simulink model "RecurDyn_Client_Block_9_1"  (R2018b)
settings: Solver=ode45  StartTime=0.0  StopTime=1.0  FixedStep=Control_timestep  RelTol=1e-3  AbsTol=1e-6
values from neighbouring files (symbols this model uses):
  Matlab_version = str2double(r_temp___(1))    [quadruped.m]
  Output_File = 'quadruped_demo1'    [quadruped.m]
  Output_file_n = r_temp___(2)    [quadruped.m]
  Plant_inputs_num = r_temp___(1)    [quadruped.m]
  Plant_outputs_num = r_temp___(1)    [quadruped.m]
  RecurDyn = 'C:\Program Files\FunctionBay, Inc\RecurDyn V9R1\Bin\'    [quadruped.m]
  RecurDyn_controltimestep = 1.e-003    (= 0.001)    [quadruped.m]
  RecurDyn_model = 'quadruped_demo1'    [quadruped.m]
  RecurDyn_model_n = r_temp___(2)    [quadruped.m]
settings Model: ExtModeTrigMode=oneshot  ExtModeArmWhenConnect=off  Creator=hgildong  LastModifiedBy=ahl19
settings SolverCC: AutoScaleAbsTol=off
settings DataIOCC: SaveFormat=Array  SignalLoggingSaveFormat=ModelDataLogs
settings OptimizationCC: BooleanDataType=off  ExpressionDepthLimit=2147483647  InitFltsAndDblsToZero=on  LifeSpan=inf
settings DebuggingCC: SaveWithParameterizedLinksMsg=none  UnderspecifiedInitializationDetection=Classic  MergeDetectMultiDrivingBlocksExec=none  SignalResolutionControl=TryResolveAllWithWarning  MultiTaskDSMMsg=warning  MultiTaskCondExecSysMsg=none  FcnCallInpInsideContextMsg=warning  StateNameClashWarn=warning  SFUnexpectedBacktrackingDiag=warning  SFNoUnconditionalDefaultTransitionDiag=warning  SFExecutionAtInitializationDiag=none
settings HardwareCC: ProdBitPerPointer=32  ProdBitPerSizeT=32  ProdBitPerPtrDiffT=32  ProdLargestAtomicFloat=None  ProdIntDivRoundTo=Undefined  ProdEndianess=Unspecified  ProdWordSize=32  ProdHWDeviceType=32-bit Generic  TargetUnknown=on
settings ModelReferenceCC: PropagateSignalLabelsOutOfModel=off
settings SFSimCC: SimUseLocalCustomCode=off
settings RTWCC: TemplateMakefile=grt_unix.tmf  RTWUseLocalCustomCode=off
settings CodeAppCC: StateflowObjectComments=on
settings GRTTargetCC: TargetFcnLib=ansi_tfl_tmw.mat  TargetLangStandard=C89/C90 (ANSI)  ModelReferenceCompliant=off  GeneratePreprocessorConditionals=Disable all  CombineOutputUpdateFcns=off  MatFileLogging=off  GRTInterface=on
settings ConfigComp: CovMetricSettings=dw  CovHtmlReporting=on  CovSaveCumulativeToWorkspaceVar=on  CovSaveSingleToWorkspaceVar=on  CovExternalEMLEnable=off

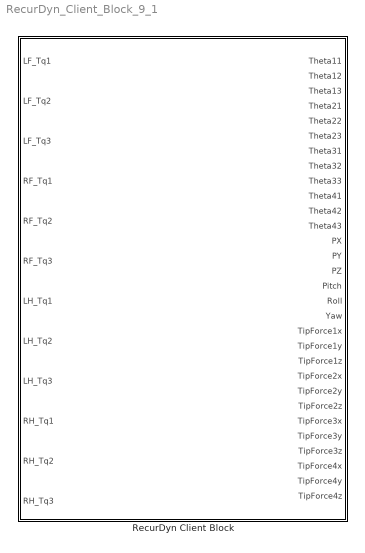
== system RecurDyn_Client_Block_9_1 ==
  RecurDyn Client Block : Subsystem
      mask Display: image(imread('RecurDyn_IF3x_Client.jpg'))

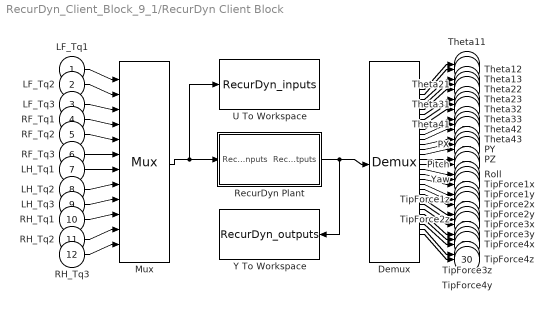
== system RecurDyn_Client_Block_9_1/RecurDyn Client Block ==
  LF_Tq1 : Inport
  LF_Tq2 : Inport  Port=2
  LF_Tq3 : Inport  Port=3
  RF_Tq1 : Inport  Port=4
  RF_Tq2 : Inport  Port=5
  RF_Tq3 : Inport  Port=6
  LH_Tq1 : Inport  Port=7
  LH_Tq2 : Inport  Port=8
  LH_Tq3 : Inport  Port=9
  RH_Tq1 : Inport  Port=10
  RH_Tq2 : Inport  Port=11
  RH_Tq3 : Inport  Port=12
  Demux : Demux  Outputs=30
  Mux : Mux  Inputs=12
  RecurDyn Plant : Subsystem  mask(Recurdyn/Plant){RecurDyn_model_name=RecurDyn_model, Output_File_Name_=Output_File, RecurDyn_=RecurDyn, Matlab_version_=Matlab_version, RecurDyn_controltimestep_=RecurDyn_controltimestep, RecurDyn_step_=100, Waitingtime=1000, RecurDyn_static_=off, RecurDyn_show_=on, RecurDyn_ani_=on, Create_Output_Folder_=off}
      mask prompts: Output_File_Name_ "Output File Name"; RecurDyn_ "RecurDyn_install_directory"; Matlab_version_ "Matlab version"; RecurDyn_controltimestep_ "Sampling period"; RecurDyn_step_ "RecurDyn_step"; Waitingtime "Waiting time"; RecurDyn_static_ "Static analysis"; RecurDyn_show_ "RecurDyn_show"; RecurDyn_ani_ "RecurDyn_animation"; Create_Output_Folder_ "Create Output Folder"
      mask help:
      | Simulate any Recurdyn Dynamics Model in Recurdyn/Solver
      | Plant inputs and Plant outputs are transfered every sampling time
      | Here, sampling time is determined by sampling period (Control time step)
      mask Display: disp( 'Dynamic Model' )
  U To Workspace : ToWorkspace  VariableName=RecurDyn_inputs
  Y To Workspace : ToWorkspace  VariableName=RecurDyn_outputs
  "Theta11   " : Outport
  "Theta12   " : Outport  Port=2
  "Theta13   " : Outport  Port=3
  "Theta21   " : Outport  Port=4
  "Theta22   " : Outport  Port=5
  "Theta23   " : Outport  Port=6
  "Theta31   " : Outport  Port=7
  "Theta32   " : Outport  Port=8
  "Theta33   " : Outport  Port=9
  "Theta41   " : Outport  Port=10
  "Theta42   " : Outport  Port=11
  "Theta43   " : Outport  Port=12
  "PX        " : Outport  Port=13
  "PY        " : Outport  Port=14
  "PZ        " : Outport  Port=15
  "Pitch     " : Outport  Port=16
  "Roll      " : Outport  Port=17
  "Yaw       " : Outport  Port=18
  TipForce1x : Outport  Port=19
  TipForce1y : Outport  Port=20
  TipForce1z : Outport  Port=21
  TipForce2x : Outport  Port=22
  TipForce2y : Outport  Port=23
  TipForce2z : Outport  Port=24
  TipForce3x : Outport  Port=25
  TipForce3y : Outport  Port=26
  TipForce3z : Outport  Port=27
  TipForce4x : Outport  Port=28
  TipForce4y : Outport  Port=29
  TipForce4z : Outport  Port=30
  wires:
  RecurDyn Plant/1(RecurDyn_outputs) -> Demux/1, Y To Workspace/1
  Mux/1 -> RecurDyn Plant/1(" RecurDyn_inputs"), U To Workspace/1
  Demux/1 -> "Theta11   "/1
  Demux/2 -> "Theta12   "/1
  Demux/3 -> "Theta13   "/1
  Demux/4 -> "Theta21   "/1
  Demux/5 -> "Theta22   "/1
  Demux/6 -> "Theta23   "/1
  Demux/7 -> "Theta31   "/1
  Demux/8 -> "Theta32   "/1
  Demux/9 -> "Theta33   "/1
  Demux/10 -> "Theta41   "/1
  Demux/11 -> "Theta42   "/1
  Demux/12 -> "Theta43   "/1
  Demux/13 -> "PX        "/1
  Demux/14 -> "PY        "/1
  Demux/15 -> "PZ        "/1
  Demux/16 -> "Pitch     "/1
  Demux/17 -> "Roll      "/1
  Demux/18 -> "Yaw       "/1
  Demux/19 -> TipForce1x/1
  Demux/20 -> TipForce1y/1
  Demux/21 -> TipForce1z/1
  Demux/22 -> TipForce2x/1
  Demux/23 -> TipForce2y/1
  Demux/24 -> TipForce2z/1
  Demux/25 -> TipForce3x/1
  Demux/26 -> TipForce3y/1
  Demux/27 -> TipForce3z/1
  Demux/28 -> TipForce4x/1
  Demux/29 -> TipForce4y/1
  Demux/30 -> TipForce4z/1
  LF_Tq1/1 -> Mux/1
  LF_Tq2/1 -> Mux/2
  LF_Tq3/1 -> Mux/3
  RF_Tq1/1 -> Mux/4
  RF_Tq2/1 -> Mux/5
  RF_Tq3/1 -> Mux/6
  LH_Tq1/1 -> Mux/7
  LH_Tq2/1 -> Mux/8
  LH_Tq3/1 -> Mux/9
  RH_Tq1/1 -> Mux/10
  RH_Tq2/1 -> Mux/11
  RH_Tq3/1 -> Mux/12

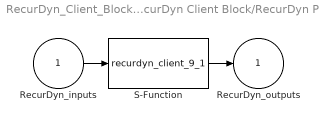
== system RecurDyn_Client_Block_9_1/RecurDyn Client Block/RecurDyn Plant ==
  " RecurDyn_inputs" : Inport
  S-Function : S-Function  FunctionName=recurdyn_client_9_1  Parameters=RecurDyn_controltimestep_,RecurDyn_model_name,RecurDyn_,RecurDyn_static_,RecurDyn_step_,RecurDyn_show_,RecurDyn_ani_,Matlab_version_,RecurDyn_model_n,Plant_inputs_num,Plant_outputs_num,Waitingtime,Create_Output_Folder_,Output_File_Name_,Output_file_n  SFunctionDeploymentMode=off  EnableBusSupport=off
  RecurDyn_outputs : Outport  InitialOutput=0
  wires:
  S-Function/1 -> RecurDyn_outputs/1
  " RecurDyn_inputs"/1 -> S-Function/1
